simulink model "ShipCoureControlModel3"  (R2021a)
settings: Solver=VariableStepAuto  StartTime=0.0  StopTime=20000  RelTol=1e-3
values from neighbouring files (symbols this model uses):
  KD = Kd_BEST    (= 0)    [PSO.m]    (also in RunningModelDemo.m = 2.5108)
  KI = Ki_BEST    (= 0)    [PSO.m]    (also in RunningModelDemo.m = 0.0983)
  KP = Kp_BEST    (= 0)    [PSO.m]    (also in RunningModelDemo.m = 1.7499)
  Tp = 10.7    [PSO.m]    (also in RunningModelDemo.m)
undefined symbols (not defined in the file or in its folder): b0, b1, b2, b3, deltaMax, K, N, PB, requiredPsi, stepTime, T1, T2, T3, useHb
settings Model: Creator=jaqbk  LastModifiedBy=Helen
settings SolverCC: AlgebraicLoopSolver=TrustRegion
settings DebuggingCC: SFMachineParentedDataDiag=warning

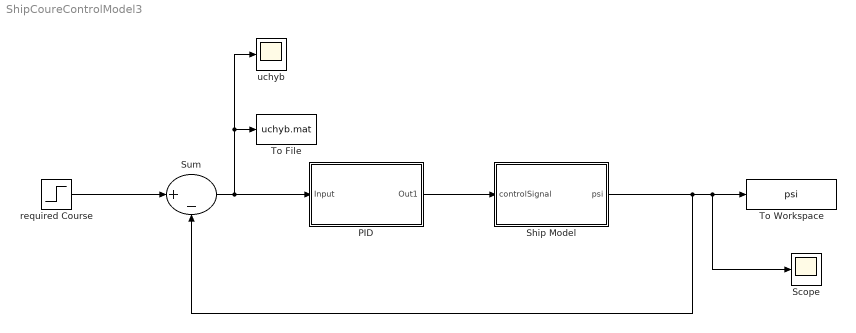
== system ShipCoureControlModel3 ==
  "PID " : Subsystem
  Scope : Scope
  Ship Model : Subsystem
  Sum : Sum  Inputs=|+-
  To File : ToFile  Filename=uchyb.mat  MatrixName=uchyb
  To Workspace : ToWorkspace  VariableName=psi  SampleTime=-1
      settings: Save2DSignal=2-D array (concatenate along first dimension)
  required Course : Step  Time=stepTime  After=requiredPsi  SampleTime=0
  uchyb : Scope
  wires:
  Ship Model/1(psi) -> Sum/2, Scope/1, To Workspace/1
  "PID "/1(Out1) -> Ship Model/1(controlSignal)
  Sum/1 -> "PID "/1(Input), To File/1, uchyb/1
  required Course/1 -> Sum/1

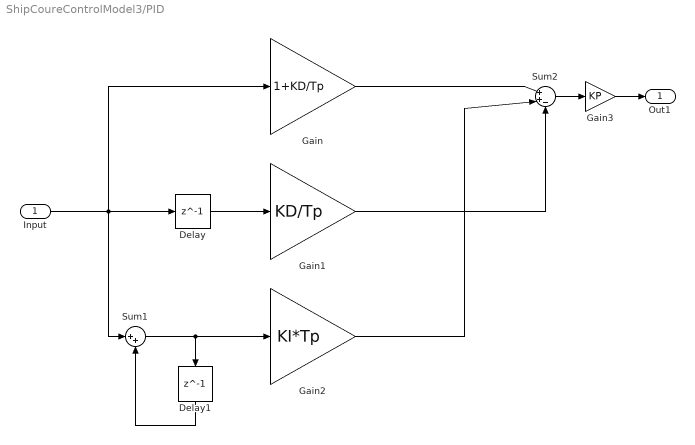
== system ShipCoureControlModel3/PID  ==
  Input : Inport
  Delay : Delay  DelayLength=1
  Delay1 : Delay  DelayLength=1
  Gain : Gain  Gain=1+KD/Tp
  Gain1 : Gain  Gain=KD/Tp
  Gain2 : Gain  Gain=KI*Tp
  Gain3 : Gain  Gain=KP
  Sum1 : Sum  Inputs=|++
  Sum2 : Sum  Inputs=|++-
  Out1 : Outport
  wires:
  Sum1/1 -> Gain2/1, Delay1/1
  Gain1/1 -> Sum2/3
  Input/1 -> Gain/1, Delay/1, Sum1/1
  Delay/1 -> Gain1/1
  Delay1/1 -> Sum1/2
  Gain3/1 -> Out1/1
  Sum2/1 -> Gain3/1
  Gain/1 -> Sum2/1
  Gain2/1 -> Sum2/2

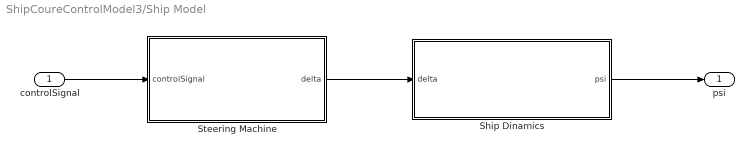
== system ShipCoureControlModel3/Ship Model ==
  controlSignal : Inport
  Ship Dinamics : Subsystem
  Steering Machine : Subsystem
  psi : Outport
  wires:
  Steering Machine/1(delta) -> Ship Dinamics/1(delta)
  controlSignal/1 -> Steering Machine/1(controlSignal)
  Ship Dinamics/1(psi) -> psi/1

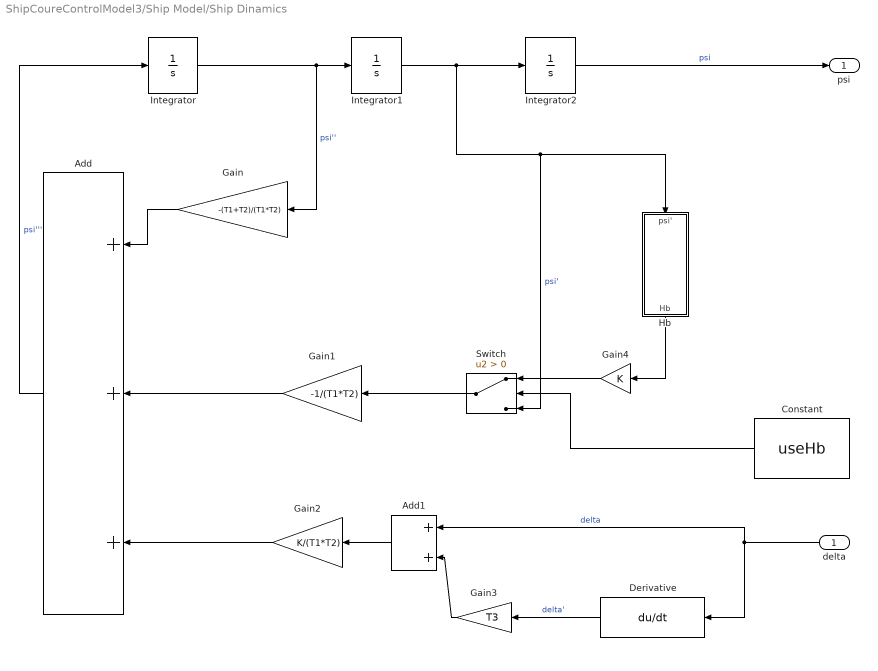
== system ShipCoureControlModel3/Ship Model/Ship Dinamics ==
  delta : Inport
  Add : Sum  Inputs=+++
  Add1 : Sum
  Constant : Constant  Value=useHb
  Derivative : Derivative
  Gain : Gain  Gain=-(T1+T2)/(T1*T2)
  Gain1 : Gain  Gain=-1/(T1*T2)
  Gain2 : Gain  Gain=K/(T1*T2)
  Gain3 : Gain  Gain=T3
  Gain4 : Gain  Gain=K
  Hb : Subsystem
  Integrator : Integrator
  Integrator1 : Integrator
  Integrator2 : Integrator
  Switch : Switch  Criteria=u2 > Threshold
  psi : Outport
  wires:
  Gain/1 -> Add/1
  Integrator1/1 -> Integrator2/1, Switch/3, Hb/1(psi')  "psi'"
  Integrator2/1 -> psi/1  "psi"
  Integrator/1 -> Gain/1, Integrator1/1  "psi''"
  Gain1/1 -> Add/2
  Add/1 -> Integrator/1  "psi'''"
  Gain2/1 -> Add/3
  delta/1 -> Add1/1, Derivative/1  "delta"
  Derivative/1 -> Gain3/1  "delta'"
  Add1/1 -> Gain2/1
  Gain3/1 -> Add1/2
  Switch/1 -> Gain1/1
  Hb/1(Hb) -> Gain4/1
  Constant/1 -> Switch/2
  Gain4/1 -> Switch/1

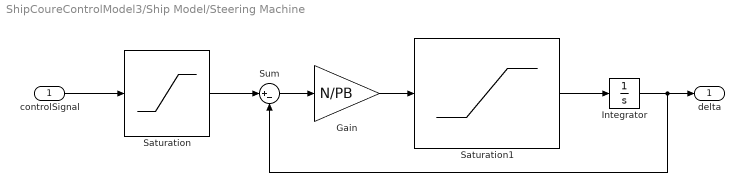
== system ShipCoureControlModel3/Ship Model/Steering Machine ==
  controlSignal : Inport
  Gain : Gain  Gain=N/PB
  Integrator : Integrator
  Saturation : Saturate  UpperLimit=deltaMax  LowerLimit=-deltaMax
  Saturation1 : Saturate  UpperLimit=N  LowerLimit=-N
  Sum : Sum  Inputs=|+-
  delta : Outport
  wires:
  controlSignal/1 -> Saturation/1
  Saturation/1 -> Sum/1
  Saturation1/1 -> Integrator/1
  Sum/1 -> Gain/1
  Gain/1 -> Saturation1/1
  Integrator/1 -> Sum/2, delta/1

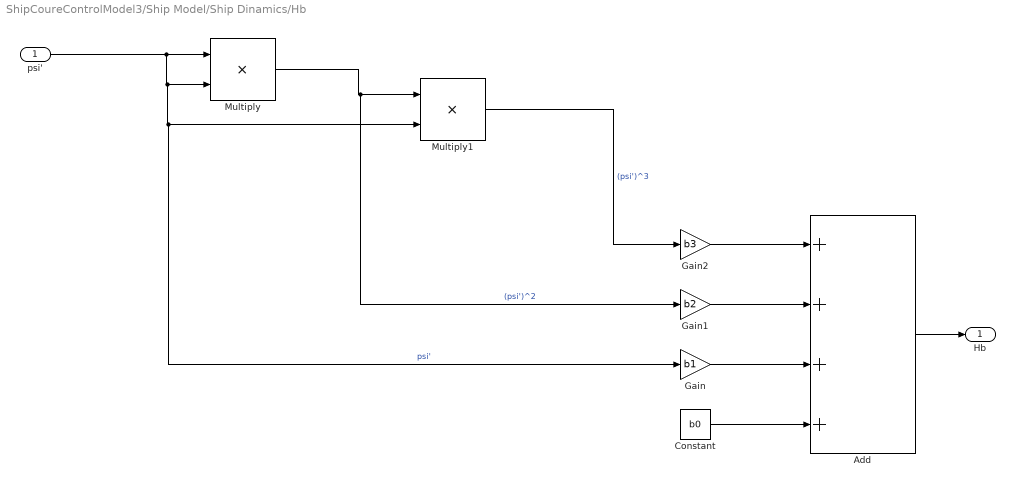
== system ShipCoureControlModel3/Ship Model/Ship Dinamics/Hb ==
  psi' : Inport
  Add : Sum  Inputs=++++
  Constant : Constant  Value=b0
  Gain : Gain  Gain=b1
  Gain1 : Gain  Gain=b2
  Gain2 : Gain  Gain=b3
  Multiply : Product  Inputs=**
  Multiply1 : Product  Inputs=**
  Hb : Outport
  wires:
  psi'/1 -> Gain/1, Multiply1/2, Multiply/2, Multiply/1  "psi'"
  Multiply/1 -> Gain1/1, Multiply1/1  "(psi')^2"
  Multiply1/1 -> Gain2/1  "(psi')^3"
  Add/1 -> Hb/1
  Constant/1 -> Add/4
  Gain/1 -> Add/3
  Gain1/1 -> Add/2
  Gain2/1 -> Add/1
